simulink model "ABSv10_01modiefied"  (R2020b)
settings: Solver=VariableStepAuto  StartTime=0.0  StopTime=100  RelTol=1e-3
undefined symbols (not defined in the file): A, c1, c2, c3, c4, Cd, d, F, H, jw, m, r, W
libraries: pid_lib x1
settings Model: Creator=K E S SRINIVAS  LastModifiedBy=K E S SRINIVAS

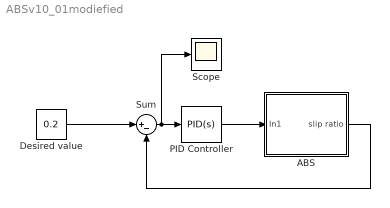
== system ABSv10_01modiefied ==
  ABS : Subsystem
  Desired value : Constant  Value=0.2
  PID Controller : pid_lib/PID Controller  Controller=PID  Form=Parallel  TimeDomain=Continuous-time  UseExternalTs=off  SampleTime=-1  IntegratorMethod=Forward Euler  FilterMethod=Forward Euler  ControllerParametersSource=internal  P=25000  I=1000000  D=10  UseFilter=on  N=100  TunerSelectOption=Transfer Function Based (PID Tuner App)  InitialConditionSource=internal  InitialConditionForIntegrator=0  InitialConditionForFilter=0  DifferentiatorICPrevScaledInput=0  ExternalReset=none  TrackingMode=off  Kt=1  LimitOutput=off  SatLimitsSource=internal  UpperSaturationLimit=inf  LowerSaturationLimit=-inf  LinearizeAsGain=on  AntiWindupMode=none  Kb=1  POutMin=[]  POutMax=[]  IOutMin=[]  IOutMax=[]  DOutMin=[]  DOutMax=[]  NOutMin=[]  NOutMax=[]  SumOutMin=[]  SumOutMax=[]  SaturationOutMin=[]  SaturationOutMax=[]  PParamMin=[]  PParamMax=[]  IParamMin=[]  IParamMax=[]  DParamMin=[]  DParamMax=[]  NParamMin=[]  NParamMax=[]  KbParamMin=[]  KbParamMax=[]  KtParamMin=[]  KtParamMax=[]  KbOutMin=[]  KbOutMax=[]  KtOutMin=[]  KtOutMax=[]  IntegratorOutMin=[]  IntegratorOutMax=[]  FilterOutMin=[]  FilterOutMax=[]  SumI1OutMin=[]  SumI1OutMax=[]  SumI2OutMin=[]  SumI2OutMax=[]  SumI3OutMin=[]  SumI3OutMax=[]  SumI4OutMin=[]  SumI4OutMax=[]  SumDOutMin=[]  SumDOutMax=[]  DifferentiatorOutMin=[]  DifferentiatorOutMax=[]  FilterDiffOutCoefMin=[]  FilterDiffOutCoefMax=[]  ReciprocalOutMin=[]  ReciprocalOutMax=[]  SumDenOutMin=[]  SumDenOutMax=[]  SumNumOutMin=[]  SumNumOutMax=[]  DivideOutMin=[]  DivideOutMax=[]  UdiffTsProdOutMin=[]  UdiffTsProdOutMax=[]  NTsProdOutMin=[]  NTsProdOutMax=[]  UintegralTsProdOutMin=[]  UintegralTsProdOutMax=[]  UngainTsProdOutMin=[]  UngainTsProdOutMax=[]  IntegratorContinuousStateAttributes=''  IntegratorStateMustResolveToSignalObject=off  IntegratorRTWStateStorageClass=Auto  FilterContinuousStateAttributes=''  FilterStateMustResolveToSignalObject=off  FilterRTWStateStorageClass=Auto  ParallelPVariant=InternalParameters  IdealPVariant=Disabled  IVariant=InternalParameters  DVariant=InternalParameters  IntegratorVariant=Continuous  SatVariant=Disabled  AWVariant=Passthrough  PCopyVariant=Disabled  TRVariant=Disabled  FdbkBlocksVariant=Forward  IdealPFdbkVariant=Disabled  SatFdbkVariant=Disabled  DerivativeFilterVariant=ContFilter  NVariant=InternalParameters  NCopyVariant=Disabled  FilterICVariant=InternalICsFilter  IntegratorICVariant=InternalICs  ExternalResetVariant=Disabled  TRSumVariant=Passthrough  SumFdbkVariant=Disabled  SumVariant=Sum_PID  TsampFilterVariant=InternalTs  TsampNgainVariant=Passthrough  TsampIntegralVariant=Passthrough  ExternalSaturationOutDataTypeStr=Inherit: Same as second input
  Scope : Scope
  Sum : Sum  Inputs=|+-
  wires:
  ABS/1(slip ratio) -> Sum/2
  Desired value/1 -> Sum/1
  PID Controller/1 -> ABS/1(In1)
  Sum/1 -> Scope/1, PID Controller/1

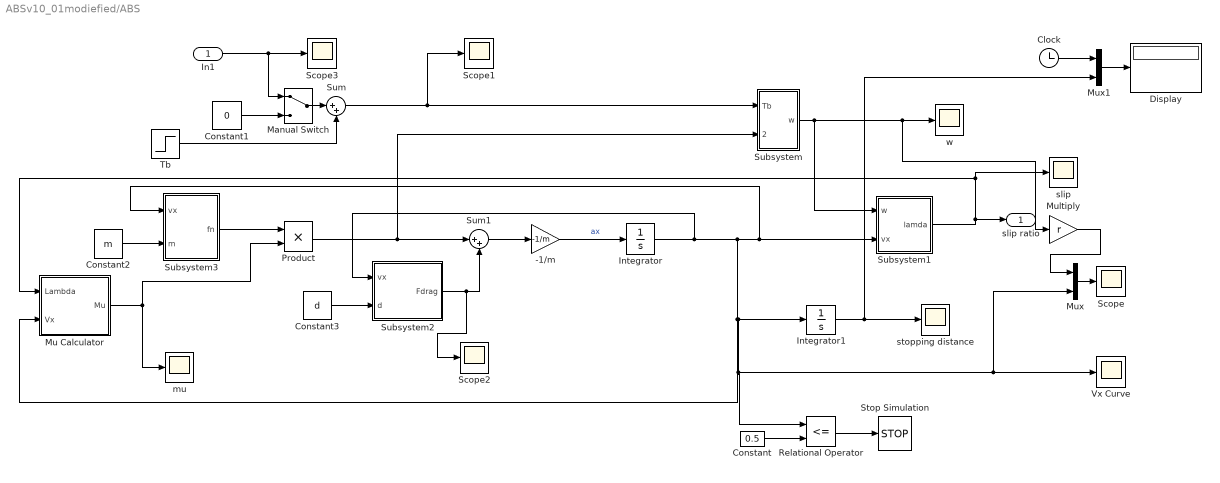
== system ABSv10_01modiefied/ABS ==
  In1 : Inport
  -1/m : Gain  Gain=-1/m
  Clock : Clock
  Constant : Constant  Value=0.5
  Constant1 : Constant  Value=0
  Constant2 : Constant  Value=m
  Constant3 : Constant  Value=d
  Display : Display
  Integrator : Integrator  InitialCondition=27.78  LimitOutput=on  LowerSaturationLimit=0
  Integrator1 : Integrator
  Manual Switch : ManualSwitch
  Mu Calculator : Subsystem
  Multiply : Gain  Gain=r
  Mux : Mux  Inputs=2
  Mux1 : Mux  Inputs=2
  Product : Product
  Relational Operator : RelationalOperator  Operator=<=  OutDataTypeStr=boolean  RndMeth=Simplest
  Scope{,1..3} (4 alike) : Scope
  Stop Simulation : Stop
  Subsystem : Subsystem
  Subsystem1 : Subsystem
  Subsystem2 : Subsystem
  Subsystem3 : Subsystem
  Sum : Sum  Inputs=|++
  Sum1 : Sum  Inputs=|++
  Tb : Step  Time=0  After=1200  SampleTime=0
  Vx Curve : Scope
  mu : Scope
  slip : Scope
  stopping distance : Scope
  w : Scope
  slip ratio : Outport
  wires:
  Mu Calculator/1(Mu) -> Product/2, mu/1
  Integrator/1 -> Mux/2, Vx Curve/1, Relational Operator/1, Integrator1/1, Mu Calculator/2(Vx), Subsystem1/2(vx), Subsystem3/1(vx), Subsystem2/1(vx)
  -1/m/1 -> Integrator/1  "ax"
  Relational Operator/1 -> Stop Simulation/1
  Constant/1 -> Relational Operator/2
  Sum/1 -> Scope1/1, Subsystem/1(Tb)
  In1/1 -> Manual Switch/1, Scope3/1
  Tb/1 -> Sum/2
  Subsystem/1(w) -> Multiply/1, w/1, Subsystem1/1(w)
  Subsystem1/1(lamda) -> slip/1, Mu Calculator/1(Lambda), slip ratio/1
  Integrator1/1 -> Mux1/2, stopping distance/1
  Mux/1 -> Scope/1
  Multiply/1 -> Mux/1
  Clock/1 -> Mux1/1
  Mux1/1 -> Display/1
  Constant1/1 -> Manual Switch/2
  Manual Switch/1 -> Sum/1
  Sum1/1 -> -1/m/1
  Subsystem2/1(Fdrag) -> Scope2/1, Sum1/2
  Constant3/1 -> Subsystem2/2(d)
  Product/1 -> Sum1/1, Subsystem/2(mu*Fn)
  Subsystem3/1(fn) -> Product/1
  Constant2/1 -> Subsystem3/2(m)

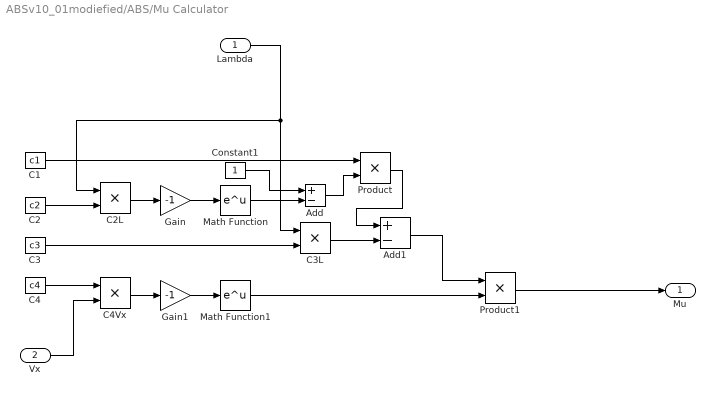
== system ABSv10_01modiefied/ABS/Mu Calculator ==
  Lambda : Inport
  Vx : Inport  Port=2
  Add : Sum  Inputs=+-
  Add1 : Sum  Inputs=+-
  C1 : Constant  Value=c1
  C2 : Constant  Value=c2
  C2L : Product
  C3 : Constant  Value=c3
  C3L : Product
  C4 : Constant  Value=c4
  C4Vx : Product
  Constant1 : Constant
  Gain : Gain  Gain=-1
  Gain1 : Gain  Gain=-1
  Math Function : Math  SaturateOnIntegerOverflow=on
  Math Function1 : Math  SaturateOnIntegerOverflow=on
  Product : Product
  Product1 : Product
  Mu : Outport
  wires:
  C2/1 -> C2L/2
  Gain/1 -> Math Function/1
  C1/1 -> Product/1
  C2L/1 -> Gain/1
  Constant1/1 -> Add/1
  Vx/1 -> C4Vx/2
  C4/1 -> C4Vx/1
  Add/1 -> Product/2
  Math Function/1 -> Add/2
  Gain1/1 -> Math Function1/1
  Math Function1/1 -> Product1/2
  C3L/1 -> Add1/2
  Lambda/1 -> C3L/1, C2L/1
  C4Vx/1 -> Gain1/1
  C3/1 -> C3L/2
  Product/1 -> Add1/1
  Add1/1 -> Product1/1
  Product1/1 -> Mu/1

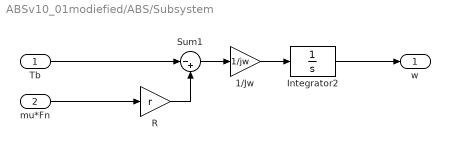
== system ABSv10_01modiefied/ABS/Subsystem ==
  Tb : Inport
  mu*Fn : Inport  Port=2
  1/Jw : Gain  Gain=1/jw
  Integrator2 : Integrator  InitialCondition=84.18  LimitOutput=on  LowerSaturationLimit=0
  R : Gain  Gain=r
  Sum1 : Sum  Inputs=|-+
  w : Outport
  wires:
  Sum1/1 -> 1/Jw/1
  Tb/1 -> Sum1/1
  Integrator2/1 -> w/1
  mu*Fn/1 -> R/1
  1/Jw/1 -> Integrator2/1
  R/1 -> Sum1/2

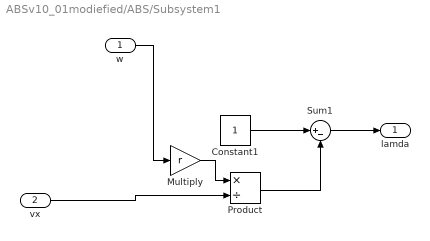
== system ABSv10_01modiefied/ABS/Subsystem1 ==
  w : Inport
  vx : Inport  Port=2
  Constant1 : Constant
  Multiply : Gain  Gain=r
  Product : Product  Inputs=*/
  Sum1 : Sum  Inputs=|+-
  lamda : Outport
  wires:
  w/1 -> Multiply/1
  Constant1/1 -> Sum1/1
  vx/1 -> Product/2
  Multiply/1 -> Product/1
  Product/1 -> Sum1/2
  Sum1/1 -> lamda/1

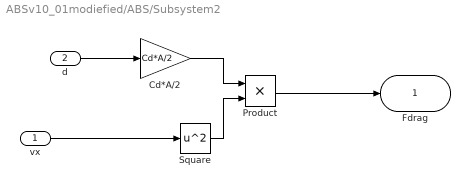
== system ABSv10_01modiefied/ABS/Subsystem2 ==
  vx : Inport
  d : Inport  Port=2
  Cd*A/2 : Gain  Gain=Cd*A/2
  Product : Product
  Square : Math  Operator=square  SaturateOnIntegerOverflow=on
  Fdrag : Outport
  wires:
  Square/1 -> Product/2
  d/1 -> Cd*A/2/1
  Cd*A/2/1 -> Product/1
  Product/1 -> Fdrag/1
  vx/1 -> Square/1

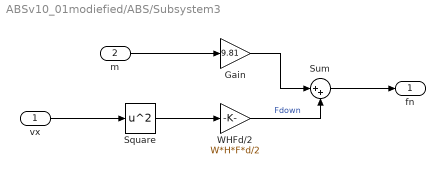
== system ABSv10_01modiefied/ABS/Subsystem3 ==
  vx : Inport
  m : Inport  Port=2
  Gain : Gain  Gain=9.81
  Square : Math  Operator=square  SaturateOnIntegerOverflow=on
  Sum : Sum  Inputs=|++
  WHFd/2 : Gain  Gain=W*H*F*d/2
  fn : Outport
  wires:
  vx/1 -> Square/1
  Square/1 -> WHFd/2/1
  Sum/1 -> fn/1
  WHFd/2/1 -> Sum/2  "Fdown"
  m/1 -> Gain/1
  Gain/1 -> Sum/1
